simulink model "ManufacturingFacility_LL"  (R2018b)
settings: Solver=VariableStepAuto  StartTime=0.0  StopTime=4000  RelTol=1e-3
undefined symbols (not defined in the file): m, n
libraries: simulink x4
settings Model: Creator=Ryan  LastModifiedBy=supriyagadigone

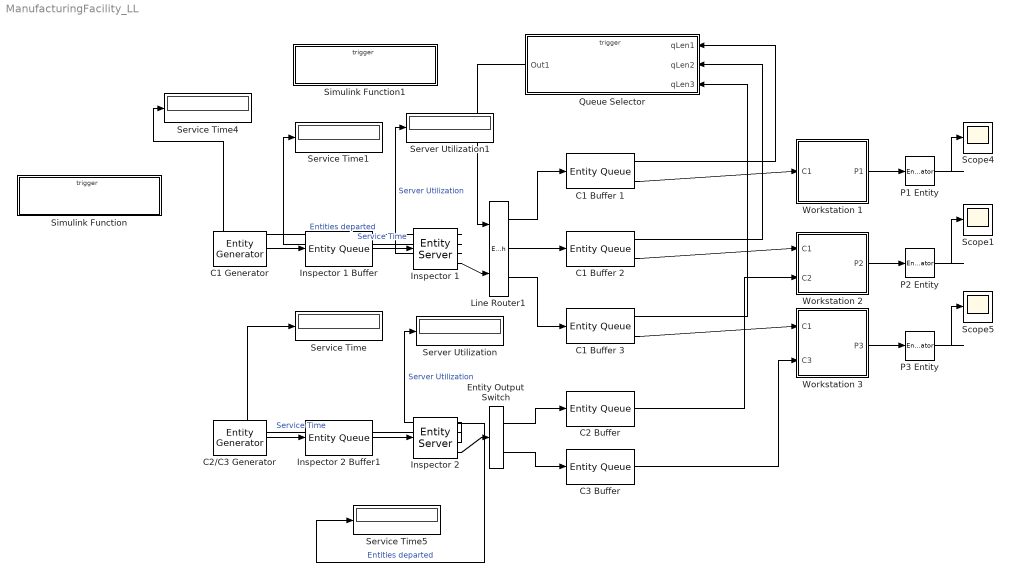
== system ManufacturingFacility_LL ==
  C1 Buffer 1 : EntityQueue  InputPortMessageModes=m  OutputPortMessageModes=n,m  Capacity=2  NumberEntitiesInBlock=on
      settings: OutputPortMap=o1,o5
  C1 Buffer 2 : EntityQueue  InputPortMessageModes=m  OutputPortMessageModes=n,m  Capacity=2  NumberEntitiesInBlock=on
      settings: OutputPortMap=o1,o5
  C1 Buffer 3 : EntityQueue  InputPortMessageModes=m  OutputPortMessageModes=n,m  Capacity=2  NumberEntitiesInBlock=on
      settings: OutputPortMap=o1,o5
  C1 Generator : EntityGenerator  OutputPortMessageModes=m  TimeSource=MATLAB action  Period=0  IntergenerationTimeAction=dt = uniformArrivalTime();  AttributeName=entityType|outputPort  AttributeInitialValue=1|1  EntityType=Structured  EntityTypeName=Entity
  C2 Buffer : EntityQueue  InputPortMessageModes=m  OutputPortMessageModes=m  Capacity=2
      settings: OutputPortMap=o5
  C2/C3 Generator : EntityGenerator  OutputPortMessageModes=m  TimeSource=MATLAB action  Period=0  IntergenerationTimeAction=dt = uniformArrivalTime();  GenerateAction=|  AttributeName=entityType|outputPort  AttributeInitialValue=1|1  EntityType=Structured  EntityTypeName=Entity
      | % Generate a random entity type corresponding
      | % To the component type
      | entity.entityType = randi([2, 3])
      | 
      | % Define the output port
      | switch entity.entityType
      |     case 2
      |         entity.outputPort = 1
      |     case 3
      |         entity.outputPort = 2
      |     otherwise
      |         error('Invalid entity type')
      | end
  C3 Buffer : EntityQueue  InputPortMessageModes=m  OutputPortMessageModes=m  Capacity=2
      settings: OutputPortMap=o5
  Entity Output Switch : EntityOutputSwitch  InputPortMessageModes=m  OutputPortMessageModes=m,m  SwitchingCriterion=From attribute  SwitchAttributeName=outputPort
  Inspector 1 : EntityServer  InputPortMessageModes=m  OutputPortMessageModes=n,n,n,m  Capacity=1  ServiceTimeSource=MATLAB action  ServiceTimeAction=|  EntryAction=|  NumberEntitiesDeparted=on  AverageWait=on  Utilization=on
      ServiceTimeAction=|
      | % dt = wblrnd(10.725, 1.096);
      | % Generate service time from uniform distribution
      | dt = uniformServiceTime();
      EntryAction=|
      | % Entity will select the shortest queue
      | pickShortestQueue();
      settings: OutputPortMap=o0,o4,o5,o9
  Inspector 1 Buffer : EntityQueue  InputPortMessageModes=m  OutputPortMessageModes=m
      settings: OutputPortMap=o5
  "Inspector 2 " : EntityServer  InputPortMessageModes=m  OutputPortMessageModes=n,n,n,m  Capacity=1  ServiceTimeSource=MATLAB action  ServiceTimeAction=|  NumberEntitiesDeparted=on  AverageWait=on  Utilization=on
      | % Depending on the type of entity
      | % Generate the appropriate service time
      | switch entity.entityType
      |     case 2
      | %         dt = wblrnd(16.0876, 1.09601);
      |           dt = uniformServiceTime();
      |     case 3
      | %         dt = exprnd(20.6328);
      |           dt = uniformServiceTime();
      |     otherwise
      |         dt = -1
      | end
      settings: OutputPortMap=o0,o4,o5,o9
  Inspector 2 Buffer1 : EntityQueue  InputPortMessageModes=m  OutputPortMessageModes=m
      settings: OutputPortMap=o5
  Line Router1 : EntityOutputSwitch  InputPortMessageModes=m,m  OutputPortMessageModes=m,m,m  NumberOutputPorts=3  SwitchingCriterion=From control port  SwitchAttributeName=QueuePath
      settings: InputPortMap=u0,u1  OutputPortMap=o0,o1,o2
  P1 Entity : EntityTerminator  InputPortMessageModes=m  NumberEntitiesArrived=on
      settings: OutputPortMap=o0
  P2 Entity : EntityTerminator  InputPortMessageModes=m  NumberEntitiesArrived=on
      settings: OutputPortMap=o0
  P3 Entity : EntityTerminator  InputPortMessageModes=m  NumberEntitiesArrived=on
      settings: OutputPortMap=o0
  Queue Selector : Subsystem  TreatAsAtomicUnit=on
  Scope1 : Scope
  Scope4 : Scope
  Scope5 : Scope
  Server Utilization : Display
  Server Utilization1 : Display
  Service Time{,1,4..5} (4 alike) : Display
      Service Time4 settings: Format=decimal (Stored Integer)
      Service Time5 settings: Format=decimal (Stored Integer)
  Simulink Function : Subsystem  TreatAsAtomicUnit=on
  Simulink Function1 : Subsystem  TreatAsAtomicUnit=on
  "Workstation 1 " : Subsystem
  Workstation 2 : Subsystem
  Workstation 3 : Subsystem
  wires:
  C1 Generator/1 -> Inspector 1 Buffer/1
  Inspector 1 Buffer/1 -> Inspector 1/1
  C1 Buffer 1/1 -> Queue Selector/1(qLen1)
  C1 Buffer 2/1 -> Queue Selector/2(qLen2)
  C1 Buffer 3/1 -> Queue Selector/3(qLen3)
  Inspector 1/4 -> Line Router1/2
  Queue Selector/1(Out1) -> Line Router1/1
  Line Router1/1 -> C1 Buffer 1/1
  Line Router1/2 -> C1 Buffer 2/1
  Line Router1/3 -> C1 Buffer 3/1
  C2/C3 Generator/1 -> Inspector 2 Buffer1/1
  Inspector 2 Buffer1/1 -> "Inspector 2 "/1
  "Inspector 2 "/4 -> Entity Output Switch/1
  Entity Output Switch/1 -> C2 Buffer/1
  Entity Output Switch/2 -> C3 Buffer/1
  P1 Entity/1 -> Scope4/1
  C1 Buffer 1/2 -> "Workstation 1 "/1(C1)
  "Workstation 1 "/1(P1) -> P1 Entity/1
  C1 Buffer 2/2 -> Workstation 2/1(C1)
  C2 Buffer/1 -> Workstation 2/2(C2)
  Workstation 2/1(P2) -> P2 Entity/1
  C1 Buffer 3/2 -> Workstation 3/1(C1)
  C3 Buffer/1 -> Workstation 3/2(C3)
  Workstation 3/1(P3) -> P3 Entity/1
  P3 Entity/1 -> Scope5/1
  P2 Entity/1 -> Scope1/1
  "Inspector 2 "/2 -> Service Time/1  "Service Time"
  "Inspector 2 "/3 -> Server Utilization/1  "Server Utilization"
  Inspector 1/2 -> Service Time1/1  "Service Time"
  Inspector 1/3 -> Server Utilization1/1  "Server Utilization"
  Inspector 1/1 -> Service Time4/1  "Entities departed"
  "Inspector 2 "/1 -> Service Time5/1  "Entities departed"

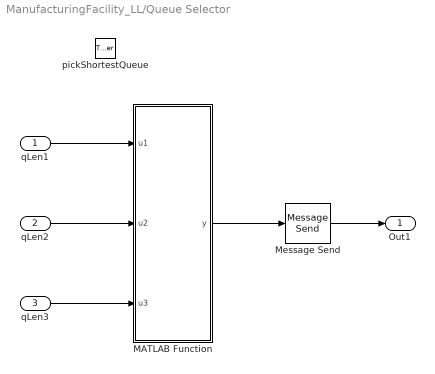
== system ManufacturingFacility_LL/Queue Selector ==
  qLen1 : Inport
  qLen2 : Inport  Port=2
  qLen3 : Inport  Port=3
  pickShortestQueue : TriggerPort  TriggerType=function-call  IsSimulinkFunction=on  FunctionName=pickShortestQueue  FunctionVisibility=scoped  VariantControl=Variant
  MATLAB Function : MATLAB Function  TreatAsAtomicUnit=on
  Message Send : MessageSend  OutputPortMessageModes=m
      settings: InputPortMap=u1
  Out1 : Outport
  wires:
  qLen1/1 -> MATLAB Function/1(u1)
  qLen2/1 -> MATLAB Function/2(u2)
  qLen3/1 -> MATLAB Function/3(u3)
  MATLAB Function/1(y) -> Message Send/1
  Message Send/1 -> Out1/1

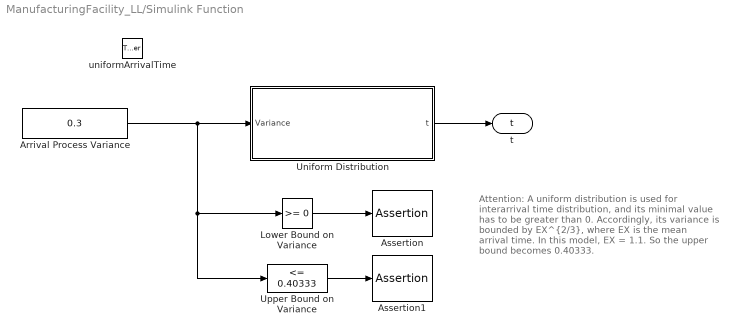
== system ManufacturingFacility_LL/Simulink Function ==
  note: Attention: A uniform distribution is used
      | for interarrival time distribution, and its
      | minimal value has to be greater than 0.
      | Accordingly, its variance is bounded by
      | EX^{2/3}, where EX is the mean arrival
      | time. In this model, EX = 1.1. So the
      | upper bound becomes 0.40333.
  uniformArrivalTime : TriggerPort  TriggerType=function-call  IsSimulinkFunction=on  FunctionName=uniformArrivalTime  VariantControl=Variant
  Arrival Process Variance : Constant  Value=0.3  SampleTime=-1
  Assertion : Assertion
  Assertion1 : Assertion
  Lower Bound on Variance : simulink/Logic and Bit Operations/Compare To Constant  relop=>=  const=0  OutDataTypeStr=uint8  ZeroCross=off
  Uniform Distribution : MATLAB Function  TreatAsAtomicUnit=on  mask{seed=12345}
  "Upper Bound on Variance " : simulink/Logic and Bit Operations/Compare To Constant  relop=<=  const=0.40333  OutDataTypeStr=uint8  ZeroCross=off
  t : ArgOut  DisableCoverage=on  ArgumentName=t
  wires:
  Uniform Distribution/1(t) -> t/1
  "Upper Bound on Variance "/1 -> Assertion1/1
  Lower Bound on Variance/1 -> Assertion/1
  Arrival Process Variance/1 -> Lower Bound on Variance/1, "Upper Bound on Variance "/1, Uniform Distribution/1(Variance)

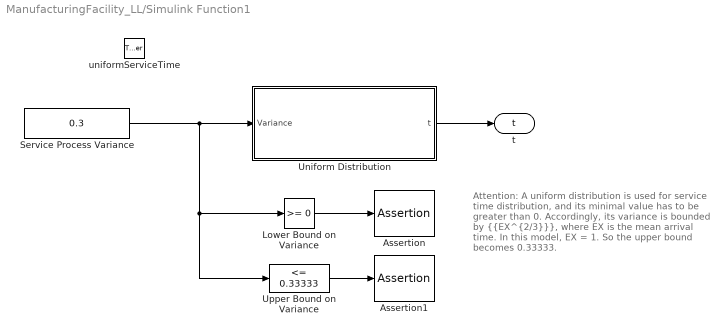
== system ManufacturingFacility_LL/Simulink Function1 ==
  note: Attention: A uniform distribution is used
      | for service time distribution, and its
      | minimal value has to be greater than 0.
      | Accordingly, its variance is bounded by
      | {{EX^{2/3}}}, where EX is the mean arrival
      | time. In this model, EX = 1. So the
      | upper bound becomes 0.33333.
  uniformServiceTime : TriggerPort  TriggerType=function-call  IsSimulinkFunction=on  FunctionName=uniformServiceTime  VariantControl=Variant
  Assertion : Assertion
  Assertion1 : Assertion
  Lower Bound on Variance : simulink/Logic and Bit Operations/Compare To Constant  relop=>=  const=0  OutDataTypeStr=uint8  ZeroCross=off
  Service Process Variance : Constant  Value=0.3  SampleTime=-1
  Uniform Distribution : MATLAB Function  TreatAsAtomicUnit=on  mask{seed=98765}
  "Upper Bound on Variance " : simulink/Logic and Bit Operations/Compare To Constant  relop=<=  const=0.33333  OutDataTypeStr=uint8  ZeroCross=off
  t : ArgOut  DisableCoverage=on  ArgumentName=t
  wires:
  Service Process Variance/1 -> Uniform Distribution/1(Variance), "Upper Bound on Variance "/1, Lower Bound on Variance/1
  Lower Bound on Variance/1 -> Assertion/1
  "Upper Bound on Variance "/1 -> Assertion1/1
  Uniform Distribution/1(t) -> t/1

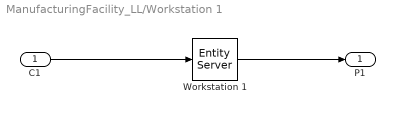
== system ManufacturingFacility_LL/Workstation 1  ==
  C1 : Inport
  Workstation 1 : EntityServer  InputPortMessageModes=m  OutputPortMessageModes=m  Capacity=1  ServiceTimeSource=MATLAB action  ServiceTimeValue=20  ServiceTimeAction=dt = exprnd(4.60442);
  P1 : Outport
  wires:
  Workstation 1/1 -> P1/1
  C1/1 -> Workstation 1/1

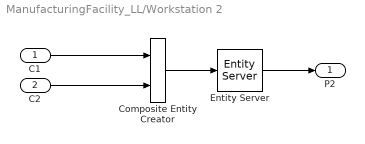
== system ManufacturingFacility_LL/Workstation 2 ==
  C1 : Inport
  C2 : Inport  Port=2
  Composite Entity Creator : CompositeEntityCreator  InputPortMessageModes=m,m  OutputPortMessageModes=m  EntityTypeName=Combined
      settings: InputPortMap=u0,u1
  Entity Server : EntityServer  InputPortMessageModes=m  OutputPortMessageModes=m  Capacity=1  ServiceTimeSource=MATLAB action  ServiceTimeValue=20  ServiceTimeAction=dt = wblrnd(10.6815, 0.922808);
  P2 : Outport
  wires:
  C2/1 -> Composite Entity Creator/2
  Composite Entity Creator/1 -> Entity Server/1
  Entity Server/1 -> P2/1
  C1/1 -> Composite Entity Creator/1

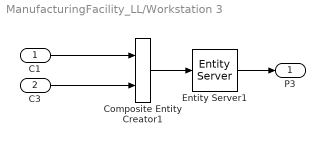
== system ManufacturingFacility_LL/Workstation 3 ==
  C1 : Inport
  C3 : Inport  Port=2
  Composite Entity Creator1 : CompositeEntityCreator  InputPortMessageModes=m,m  OutputPortMessageModes=m  EntityTypeName=Combined
      settings: InputPortMap=u0,u1
  Entity Server1 : EntityServer  InputPortMessageModes=m  OutputPortMessageModes=m  Capacity=1  ServiceTimeSource=MATLAB action  ServiceTimeValue=20  ServiceTimeAction=dt = exprnd(8.79558);
  P3 : Outport
  wires:
  Entity Server1/1 -> P3/1
  C3/1 -> Composite Entity Creator1/2
  Composite Entity Creator1/1 -> Entity Server1/1
  C1/1 -> Composite Entity Creator1/1

== matlab function ManufacturingFacility_LL/Queue Selector/MATLAB Function ==
  data: u1 input; y output; u2 input; u3 input
function y = fcn(u1, u2, u3)
%#codegen

% Identify which input index is the smallest
[~,y] = min([u1 u2 u3]);

== matlab function ManufacturingFacility_LL/Simulink Function/Uniform Distribution ==
  data: t output; Variance input; seed parameter
function t = GenInterArrivalTime(Variance, seed)
% This function generates uniformly distributed interarrival time
% distributed in [0,b] interval with the specified variance and 
% mean arrival time

persistent initialize_seed;
% Initialize the seed for the 
% first call
if(isempty(initialize_seed))
    rng(seed,'v4');
    initialize_seed = 1;
end

MeanArrivalTime = 1.1;
% The lower limit for the uniform distribution is 0;
% b is the upper limit of the uniform distribution
% for the given variance
b = 2*sqrt(3*Variance);

% Center the distribution around zero: b(rng-1/2)
% Shift the distribution to get the mean arrival time
t = b*(rand-1/2) + MeanArrivalTime;

== matlab function ManufacturingFacility_LL/Simulink Function1/Uniform Distribution ==
  data: t output; Variance input; seed parameter
function t = GenInterArrivalTime(Variance, seed)
% This function generates uniformly distributed interarrival time
% distributed in [0,b] interval with the specified variance and 
% mean arrival time

persistent initialize_seed;
% Initialize the seed for the 
% first call
if(isempty(initialize_seed))
    rng(seed,'v4');
    initialize_seed = 1;
end

MeanArrivalTime = 1.1;
% The lower limit for the uniform distribution is 0;
% b is the upper limit of the uniform distribution
% for the given variance
b = 2*sqrt(3*Variance);

% Center the distribution around zero: b(rng-1/2)
% Shift the distribution to get the mean arrival time
t = b*(rand-1/2) + MeanArrivalTime;
